simulink model "ADC_DMA_MATLAB_Statemachine"  (R2020a)
settings: Solver=VariableStepAuto  StartTime=0.0  StopTime=10.0  RelTol=1e-3
settings Model: Creator=swaga  LastModifiedBy=swaga

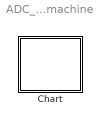
== system ADC_DMA_MATLAB_Statemachine ==
  Chart : Stateflow chart  TreatAsAtomicUnit=on

== stateflow chart ADC_DMA_MATLAB_Statemachine/Chart ==
  note: Start
  note: UART_Rx_IRQ() - Request to Send from MATLAB
  state INITIALIZE
    'ALL GLOBAL VARIABLE'
    'ADC_START'
    'UART_START'
    'DAC_START'
    'UART_Rx_INTERRUPT_START'
    'PUSH_BTN_INTERRUPT_START'
    'DMA_DONE_INTERRUPT_START'
  state ADC_SAMPLING
  state DMA_TRANSFER_TO_SRAM
    'DMA_ENABLED'
    'Total 2048 Bytes transfered'
    'DMA_DISABLED'
  note: PBTN to be pressed only once
      | PBTN flag will reset automatically after
      | data received 10 times by MATLAB
  note: push_button_IRQ()
  state RED_LED [group]
    state RED_LED_ON
    state RED_LED_OFF
  state BLUE_LED [group]
    state BLUE_LED_ON
    state BLUE_LED_OFF
    BLUE_LED_ON -> BLUE_LED_OFF : ['after (Delay_500ms)']
        | {time = 500}
  state GREEN_LED [group]
    state GREEN_LED_ON
    state GREEN_LED_OFF
    GREEN_LED_ON -> GREEN_LED_OFF : ['after (Delay_1000ms)']
        | {time = 1000}
  state UART_TRANSFER
    'transfer_SRAM_to_UART_Tx_BUFFER'
    'transfer_UART_Tx_BUFFER_TO_COMPORT'
  note: Green LED
      | Blink in every 1000ms
      | {system in ideal condition}
  note: Red LED
      | {on =DMA transfer done
      | off = UART transfer done}
  note: BLUE LED
      | {blink 3 times = matlab received data 10 times}
  state DATA_COUNTER
    'increment_COUNTER'
    count_value = count_value + 1;
    'reset_DMA_TRANSFER_DONE_FLAG'
    DMA_TRANSFER_DONE_FLAG = False;
  BLUE_LED -> ADC_SAMPLING
  (default) -> INITIALIZE
  ADC_SAMPLING -> DMA_TRANSFER_TO_SRAM [order 2] : ['at(UART_Rx_interrupt)']
      | {REQUEST_FOR_Tx_FLAG = True
      | DATA_RECEIVED_by_MATLAB_FLAG = False}
  INITIALIZE -> ADC_SAMPLING
  ADC_SAMPLING -> UART_TRANSFER [order 3] : ['at(push_button_interrupt)' ]
      | {PUSH_BTN_PRESSED_FALLING_EDGE = True
      |   DMA_TRANSFER_DONE_FLAG = True}
  GREEN_LED_OFF -> ADC_SAMPLING : ['after (green_led_action)']
      | {GREEN_LED_OFF =True}
  ADC_SAMPLING -> GREEN_LED_ON [order 1] : ['after (sampling_done_action']
      | {sampling_done = True}
  DMA_TRANSFER_TO_SRAM -> RED_LED_ON : ['after (dma_transfer_complete)']
      | {DMA_TRANSFER_DONE_FLAG = True}
  DATA_COUNTER -> BLUE_LED_ON [order 2] : ['after(data_count_done']
      | {count_value = 11}
  BLUE_LED_OFF -> BLUE_LED_ON
  DATA_COUNTER -> RED_LED_OFF [order 1] : ['after(dma_flag_reset)']
      | {DMA_TRANSFER_DONE_FLAG =False
      | delay_time_ms = 100}
